simulink model "Thermostat"  (R2023a)
settings: Solver=ode15s  StartTime=0.0  StopTime=20.0  FixedStep=0.01  RelTol=1e-3
settings Model: Creator=23208  LastModifiedBy=wkmiao

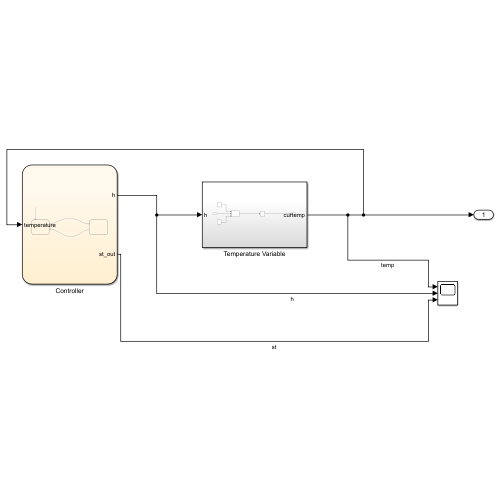
[thumbnail: Simulink's stored preview of the top-level diagram]
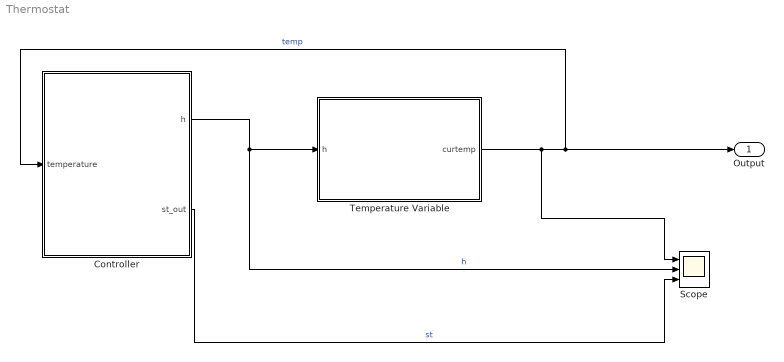
== system Thermostat ==
  Controller : Stateflow chart  TreatAsAtomicUnit=on
  Scope : Scope  NumInputPorts=3
  Temperature Variable : Subsystem
  Output : Outport
  wires:
  Temperature Variable/1(curtemp) -> Scope/1, Output/1, Controller/1(temperature)  "temp"
  Controller/1(h) -> Scope/2, Temperature Variable/1(h)  "h"
  Controller/2(st_out) -> Scope/3  "st"

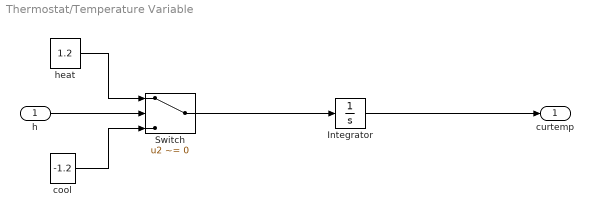
== system Thermostat/Temperature Variable ==
  h : Inport
  Integrator : Integrator  InitialCondition=22
  Switch : Switch  Criteria=u2 ~= 0  SaturateOnIntegerOverflow=off  InputSameDT=off
  cool : Constant  Value=-1.2
  heat : Constant  Value=1.2
  curtemp : Outport
  wires:
  h/1 -> Switch/2
  heat/1 -> Switch/1
  cool/1 -> Switch/3
  Integrator/1 -> curtemp/1
  Switch/1 -> Integrator/1

== stateflow chart Thermostat/Controller ==
  settings: updateMethod=CONTINUOUS
  state cooling
    du:
    h = 0;
    st_dot = 1;
    st_out = st;
  state heating
    du:
    h = 1;
    st_dot = 1;
    st_out = st;
  (default) -> cooling : {st=Tc}
  cooling -> heating : [temperature<=20&st>=Tc]{st=0}
  heating -> cooling : [temperature>=20&st>=Th]{st=0}
  data: h output double; temperature input double; Th local double =5; Tc local double =5; st local double; st_out output double
  data st settings: updateMethod=SF_CONTINUOUS_TIME_DATA
